simulink model "flightControl"  (R2015b)
settings: Solver=FixedStepDiscrete  StartTime=0.0  StopTime=inf  FixedStep=1/1000  RelTol=1e-3
libraries: simulink x1, embdlinuxlib x1, quadLibrary x1
settings Model: SimulationMode=external  ExtModeEnableFloating=off  ExtModeTrigDuration=100  Creator=Nik Descher  LastModifiedBy=Nik Descher
settings DataIOCC: LimitDataPoints=off
settings OptimizationCC: OptimizeModelRefInitCode=on  LifeSpan=1
settings HardwareCC: ProdBitPerPointer=32  ProdLargestAtomicInteger=Long  ProdLargestAtomicFloat=Double  ProdWordSize=32  ProdHWDeviceType=ARM Compatible->ARM Cortex
settings RTWCC: SystemTargetFile=realtime.tlc  GenerateMakefile=off  TemplateMakefile=realtime.tmf  Description=Run on Target Hardware  RTWVerbose=off
settings STFCustomTargetCC: TargetLibSuffix=.a  GenerateSampleERTMain=on  ConcurrentExecutionCompliant=off  GeneratePreprocessorConditionals=Use local settings  ERTCustomFileBanners=on  SupportNonInlinedSFcns=off  SupportVariableSizeSignals=on  MATLABClassNameForMDSCustomization=Simulink.SoftwareTarget.ERTCustomization  CPPClassGenCompliant=off  GRTInterface=off  SystemTargetFile=realtime.tlc
settings ERTTargetCC: GenerateSampleERTMain=on  ParMdlRefBuildCompliant=off  CompOptLevelCompliant=off  ConcurrentExecutionCompliant=off  CombineOutputUpdateFcns=off  ERTFirstTimeCompliant=off  SupportContinuousTime=on  SupportVariableSizeSignals=on  ModelStepFunctionPrototypeControlCompliant=off  CPPClassGenCompliant=off  UseToolchainInfoCompliant=off  ExtModeMexArgs='192.168.1.248' 0 17724  ERTSrcFileBannerTemplate=realtime_code_template.cgt  ERTHdrFileBannerTemplate=realtime_code_template.cgt  ERTDataSrcFileTemplate=realtime_code_template.cgt  ERTDataHdrFileTemplate=realtime_code_template.cgt  ERTCustomFileTemplate=realtime_file_process.tlc

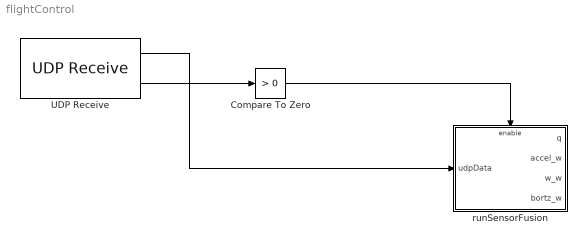
== system flightControl ==
  Compare To Zero : simulink/Logic and Bit Operations/Compare To Zero  relop=>  OutDataTypeStr=boolean
  UDP Receive : embdlinuxlib/UDP Receive  localURL='0.0.0.0'  localPort=25000  remoteURL='0.0.0.0'  remotePort=-1  recvBufferSize=8192  signalDatatype=single  dims=31  isVarSize=off  showBlockingTime=off  blockingTime=0  sampletime=1/1000  blockPlatform=Raspberry Pi
  runSensorFusion : Subsystem  TreatAsAtomicUnit=on
  wires:
  UDP Receive/1 -> runSensorFusion/1(udpData)
  UDP Receive/2 -> Compare To Zero/1
  Compare To Zero/1 -> runSensorFusion/Enable

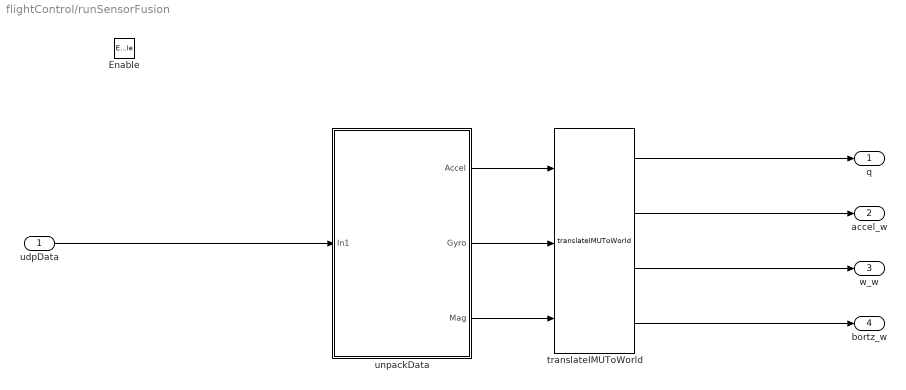
== system flightControl/runSensorFusion ==
  udpData : Inport
  Enable : EnablePort
  translateIMUToWorld : quadLibrary/translateIMUToWorld
  unpackData : Subsystem
  q : Outport
  accel_w : Outport  Port=2
  w_w : Outport  Port=3
  bortz_w : Outport  Port=4
  wires:
  udpData/1 -> unpackData/1(In1)
  unpackData/1(Accel) -> translateIMUToWorld/1
  unpackData/2(Gyro) -> translateIMUToWorld/2
  unpackData/3(Mag) -> translateIMUToWorld/3
  translateIMUToWorld/1 -> q/1
  translateIMUToWorld/2 -> accel_w/1
  translateIMUToWorld/3 -> w_w/1
  translateIMUToWorld/4 -> bortz_w/1

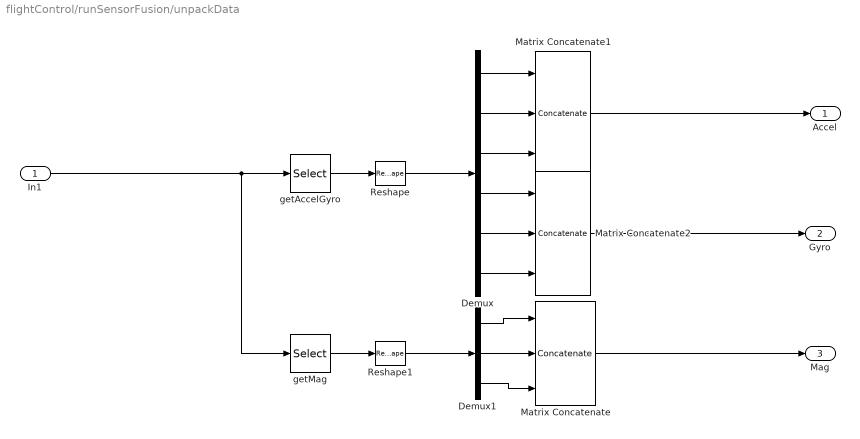
== system flightControl/runSensorFusion/unpackData ==
  In1 : Inport
  Demux : Demux  Outputs=6
  Demux1 : Demux  Outputs=3
  Matrix Concatenate : Concatenate  NumInputs=3  Mode=Multidimensional array
  Matrix Concatenate1 : Concatenate  NumInputs=3  Mode=Multidimensional array
  Matrix Concatenate2 : Concatenate  NumInputs=3  Mode=Multidimensional array
  Reshape : Reshape
  Reshape1 : Reshape
  getAccelGyro : Selector  InputPortWidth=31  IndexOptions=Index vector (dialog)  Indices=1:24  OutputSizes=1
  getMag : Selector  InputPortWidth=31  IndexOptions=Index vector (dialog)  Indices=25:30  OutputSizes=1
  Accel : Outport
  Gyro : Outport  Port=2
  Mag : Outport  Port=3
  wires:
  In1/1 -> getMag/1, getAccelGyro/1
  getMag/1 -> Reshape1/1
  Reshape1/1 -> Demux1/1
  Demux1/2 -> Matrix Concatenate/2
  Demux1/1 -> Matrix Concatenate/1
  Demux1/3 -> Matrix Concatenate/3
  Demux/2 -> Matrix Concatenate1/2
  Demux/3 -> Matrix Concatenate1/3
  Demux/1 -> Matrix Concatenate1/1
  Demux/4 -> Matrix Concatenate2/1
  Demux/5 -> Matrix Concatenate2/2
  Reshape/1 -> Demux/1
  getAccelGyro/1 -> Reshape/1
  Demux/6 -> Matrix Concatenate2/3
  Matrix Concatenate2/1 -> Gyro/1
  Matrix Concatenate/1 -> Mag/1
  Matrix Concatenate1/1 -> Accel/1
